simulink model "LCC_AngleControl"  (R2025b)
settings: Solver=FixedStepAuto  StartTime=0.0  StopTime=10.0  FixedStep=.05  RelTol=1e-3
libraries: simulink_extras x1, dspstat3 x1
settings Model: Creator=scb548  LastModifiedBy=scb548
settings OptimizationCC: ZeroExternalMemoryAtStartup=off  ZeroInternalMemoryAtStartup=off
settings RTWCC: SystemTargetFile=rtmaps.tlc  TemplateMakefile=rtmaps_default_tmf  PostCodeGenCommand=rtmaps_post_code_generation(buildInfo)  RetainRTWFile=on  TargetLang=C++  GPUComputeCapability=3.5  Description=Generate an RTMaps component embedding the model
settings STFCustomTargetCC: SystemTargetFile=rtmaps.tlc  TargetLangStandard=C++11 (ISO)  ModelReferenceCompliant=off  CombineOutputUpdateFcns=on  CodeInterfacePackaging=C++ class  SubcomponentCodeInterfacePackaging=C++ class  CPPClassGenCompliant=on  GRTInterface=off  RTMAPS_BOARD=ubuntu2204_x86_64  CustomFileTemplate=rtmaps_file_process.tlc  RTMaps_MultiInstanceCode=1  RTMaps_GRTInterface=0  RTMAPS_ARCH=x86_64  RTMAPS_OS=ubuntu2204  RTMaps_CombineOutputUpdateFcns=1  RTMaps_GenerateAllocFcn=0  DisplayOptimOptions=off  RTMaps_GenerateERTSFunction=0  RTMaps_IntegerCode=0  RTMaps_MatFileLogging=0  RTMAPS_SDKDIR=/opt/rtmaps
settings GRTTargetCC: TargetLangStandard=C++11 (ISO)  ModelReferenceCompliant=off  ParMdlRefBuildCompliant=off  CompOptLevelCompliant=off  MatFileLogging=off  CodeInterfacePackaging=C++ class  SubcomponentCodeInterfacePackaging=C++ class  UseToolchainInfoCompliant=off

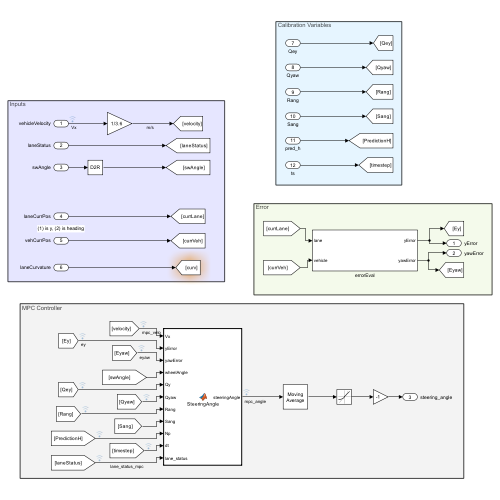
[thumbnail: Simulink's stored preview of the top-level diagram]
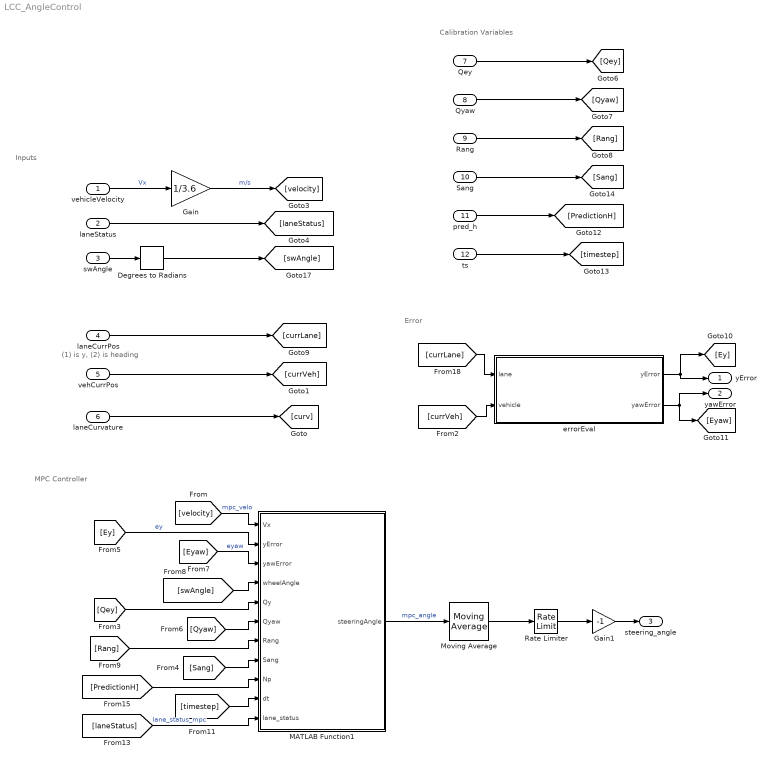
== system LCC_AngleControl ==
  note: Error
  note: (1) is y, (2) is heading
  note: Inputs
  note: Calibration Variables
  note: MPC Controller
  vehicleVelocity : Inport
  laneStatus : Inport  Port=2
  swAngle : Inport  Port=3
  laneCurrPos : Inport  Port=4
  vehCurrPos : Inport  Port=5
  laneCurvature : Inport  Port=6
  Qey : Inport  Port=7
  Qyaw : Inport  Port=8
  Rang : Inport  Port=9
  Sang : Inport  Port=10
  pred_h : Inport  Port=11
  ts : Inport  Port=12
  Degrees to Radians : simulink_extras/Transformations/Degrees to Radians
  Gain : Gain  Gain=1/3.6
  Gain1 : Gain  Gain=-1
  MATLAB Function1 : MATLAB Function  TreatAsAtomicUnit=on  SystemSampleTime=.05
  Moving Average : dspstat3/Moving Average  Method=Sliding window  ForgettingFactorPort=off  SpecifyWindowLength=on  WindowLength=4  OverlapLength=3  AllowArbitraryInputLength=off  ForgettingFactor=0.9  SimulateUsing=Interpreted execution
  Rate Limiter : RateLimiter  SampleTimeMode=inherited
  errorEval : Subsystem
  yError : Outport
  yawError : Outport  Port=2
  steering_angle : Outport  Port=3
  wires:
  laneStatus/1 -> [laneStatus]
  vehCurrPos/1 -> [currVeh]
  [currLane] -> errorEval/1(lane)
  [Sang] -> MATLAB Function1/8(Sang)
  vehicleVelocity/1 -> Gain/1  "Vx"
  [swAngle] -> MATLAB Function1/4(wheelAngle)
  laneCurvature/1 -> [curv]
  errorEval/2(yawError) -> yawError/1, [Eyaw]
  [Ey] -> MATLAB Function1/2(yError)  "ey"
  [Qey] -> MATLAB Function1/5(Qy)
  [velocity] -> MATLAB Function1/1(Vx)  "mpc_velo"
  Degrees to Radians/1 -> [swAngle]
  [PredictionH] -> MATLAB Function1/9(Np)
  swAngle/1 -> Degrees to Radians/1
  Gain/1 -> [velocity]  "m/s"
  [Eyaw] -> MATLAB Function1/3(yawError)  "eyaw"
  [Rang] -> MATLAB Function1/7(Rang)
  [currVeh] -> errorEval/2(vehicle)
  MATLAB Function1/1(steeringAngle) -> Moving Average/1  "mpc_angle"
  errorEval/1(yError) -> [Ey], yError/1
  [Qyaw] -> MATLAB Function1/6(Qyaw)
  [timestep] -> MATLAB Function1/10(dt)
  laneCurrPos/1 -> [currLane]
  [laneStatus] -> MATLAB Function1/11(lane_status)  "lane_status_mpc"
  Qyaw/1 -> [Qyaw]
  Qey/1 -> [Qey]
  Rang/1 -> [Rang]
  Sang/1 -> [Sang]
  pred_h/1 -> [PredictionH]
  ts/1 -> [timestep]
  Rate Limiter/1 -> Gain1/1
  Moving Average/1 -> Rate Limiter/1
  Gain1/1 -> steering_angle/1

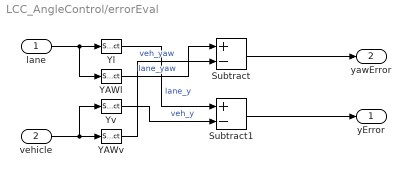
== system LCC_AngleControl/errorEval ==
  lane : Inport
  vehicle : Inport  Port=2
  Subtract : Sum  Inputs=+-
  Subtract1 : Sum  Inputs=+-
  YAWl : Selector  InputPortWidth=2  IndexOptions=Index vector (dialog)  Indices=1  OutputSizes=1
  YAWv : Selector  InputPortWidth=2  IndexOptions=Index vector (dialog)  Indices=1  OutputSizes=1
  Yl : Selector  InputPortWidth=2  IndexOptions=Index vector (dialog)  Indices=2  OutputSizes=1
  Yv : Selector  InputPortWidth=2  IndexOptions=Index vector (dialog)  Indices=2  OutputSizes=1
  yError : Outport
  yawError : Outport  Port=2
  wires:
  YAWl/1 -> Subtract/1  "lane_yaw"
  YAWv/1 -> Subtract/2  "veh_yaw"
  Yl/1 -> Subtract1/1  "lane_y"
  lane/1 -> YAWl/1, Yl/1
  Yv/1 -> Subtract1/2  "veh_y"
  vehicle/1 -> Yv/1, YAWv/1
  Subtract/1 -> yawError/1
  Subtract1/1 -> yError/1

== matlab function LCC_AngleControl/MATLAB Function1 ==
  data: Vx input; steeringAngle output; yError input; yawError input; wheelAngle input; Qy input; Qyaw input; Rang input; Sang input; Np input; dt input; lane_status input
function steeringAngle = SteeringAngle(Vx, yError, yawError, wheelAngle, Qy, Qyaw, Rang, Sang, Np, dt, lane_status)

    persistent u0
    if isempty(u0)
        u0 = wheelAngle*ones(Np, 1);
    end

    if lane_status == 0
        steeringAngle = u0(1);
    else
    
        if Vx == 0
            Vx = .001;
        end
        
        if Vx > 8.9
            Vx = 8.9;
        end
    
        % Weight matrices
        Q = diag([Qyaw, Qy]);  % Higher weight on yaw and y errors
        R = Rang;            % Penalize steering angle magnitude
        S = Sang;             % Penalize steering angle rate
        
        % Vehicle parameters (Slide 42)
        m = 2721.6;
        Jz = 2624;
        lf = 1.5;
        lr = 1.5;
        Cf = 12000;
        Cr = 20000;
        
        % Continuous model (Slide 42)
        A = [-(Cf+Cr)/(m*Vx), -Vx - (Cf*lf - Cr*lr)/(m*Vx), 0, 0;
             -(Cf*lf - Cr*lr)/(Jz*Vx), -(Cf*lf^2 + Cr*lr^2)/(Jz*Vx), 0, 0;
             0, 1, 0, 0;
             1, 0, Vx, 0];
        B = [Cf/m; (Cf*lf)/Jz; 0; 0];
        C = [0 0 1 0; 0 0 0 1]; % Extract yaw and lateral position
        
        % Discretize
        Ad = eye(4) + A * dt;
        Bd = B * dt;
        
        % Initial state
        x0 = [0; 0; yawError; yError];
        
        % Preallocate F and G
        F = [];
        G = [];
    
        for i = 1:Np
            Ai = Ad^i;
            F = [F; C * Ai];
            
            Gi = zeros(2, Np);
            for j = 1:i
                Gi(:, j) = C * Ad^(i-j) * Bd;
            end
            G = [G; Gi];
        end
        
        % Construct reference vector
        yref = zeros(2*Np, 1);
        
        % Construct weight matrices
        Qblk = kron(eye(Np), Q);
        Rblk = kron(eye(Np), R);
        Sblk = kron(eye(Np-1), S);
        
        % Construct delta rate penalty matrix T
        T = zeros(Np - 1, Np);
        for i = 1:Np - 1
            T(i, i) = -1;
            T(i, i + 1) = 1;
        end
        
        % Cost matrices
        H = G' * Qblk * G + Rblk + T' * Sblk * T;
        f = G' * Qblk * (F * x0 - yref);

        % Solve with quadprog
        delta = quadprog(2*H,2*f,[],[],[],[],[],[],u0,optimoptions('quadprog','Algorithm','active-set'));

        steeringAngle = delta(1);
    
        u0 = delta;
    end
end
